simulink model "triJunction_21_"  (R2015a)
settings: Solver=FixedStepDiscrete  StartTime=0.0  StopTime=1.0  FixedStep=1.0  RelTol=1e-3
libraries: taXlibrary x10
settings Model: Creator=emmert  LastModifiedBy=thomas
settings DataIOCC: SignalLoggingSaveFormat=ModelDataLogs
settings OptimizationCC: ExpressionDepthLimit=2147483647
settings DebuggingCC: UnderspecifiedInitializationDetection=Classic  MergeDetectMultiDrivingBlocksExec=none  SolverPrmCheckMsg=warning  FcnCallInpInsideContextMsg=EnableAllAsWarning  StateNameClashWarn=warning
settings GRTTargetCC: CombineOutputUpdateFcns=off  GRTInterface=on

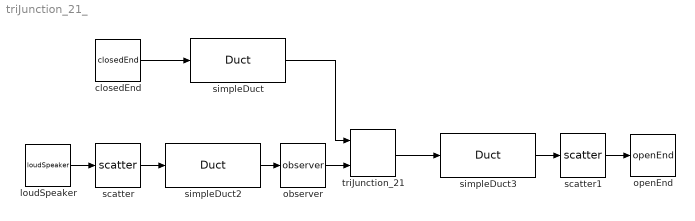
== system triJunction_21_ ==
  closedEnd : taXlibrary/closedEnd  element=closedEnd  loc=Upstream  A=1  Mach=0.1  rho=1.2  c=100
  loudSpeaker : taXlibrary/loudSpeaker  element=loudSpeaker  loc=Upstream  Amp=1  A=1.4  Mach=0.1  rho=1.2  c=100
      settings: AttributesFormatString=%<Amp> m/s
  observer : taXlibrary/observer  element=observer  property=p_u
  openEnd : taXlibrary/openEnd  element=openEnd  loc=Downstream  A=1  Mach=0.1  rho=1.2  c=100
  scatter : taXlibrary/scatter  element=scatteringDummy  loc=Upstream
  scatter1 : taXlibrary/scatter  element=scatteringDummy  loc=Downstream
  simpleDuct : taXlibrary/Duct  element=Duct  order=3  minres=40  l=0.25  sensorPositions=[]
      settings: AttributesFormatString=%<l> m
  simpleDuct2 : taXlibrary/Duct  element=Duct  order=3  minres=40  l=0.25  sensorPositions=[]
      settings: AttributesFormatString=%<l> m
  simpleDuct3 : taXlibrary/Duct  element=Duct  order=3  minres=40  l=0.25  sensorPositions=[]
      settings: AttributesFormatString=%<l> m
  triJunction_21 : taXlibrary/triJunction_21  element=triJunction_21  zetai=0  zetaj=0  A=1  rho=1.2  c=100
  wires:
  loudSpeaker/1 -> scatter/1
  scatter/1 -> simpleDuct2/1
  simpleDuct2/1 -> observer/1
  simpleDuct3/1 -> scatter1/1
  scatter1/1 -> openEnd/1
  observer/1 -> triJunction_21/2
  closedEnd/1 -> simpleDuct/1
  simpleDuct/1 -> triJunction_21/1
  triJunction_21/1 -> simpleDuct3/1
